simulink model "Simple"  (Simulink 7.4)
settings: Solver=ode45  StartTime=0.0  StopTime=80  RelTol=1e-3
settings Model: Creator=Lluís  LastModifiedBy=Lluís

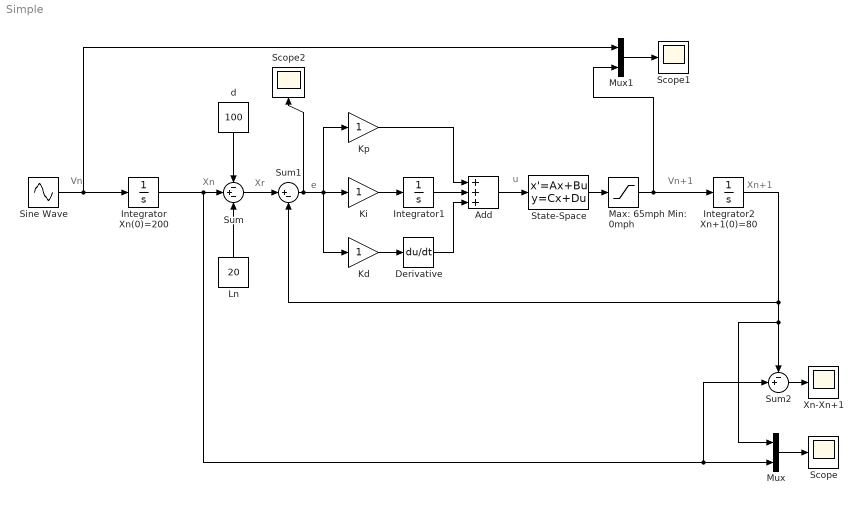
== system Simple ==
  note: Vn
  note: Xn
  note: Xr
  note: e
  note: u
  note: Vn+1
  note: Xn+1
  Add : Sum  Inputs=+++  OutDataType=fixdt(1, 16)  OutScaling=2^-10
  Derivative : Derivative
  Integrator Xn(0)=200 : Integrator  InitialCondition=200
  Integrator1 : Integrator
  Integrator2 Xn+1(0)=80 : Integrator  InitialCondition=80
  Kd : Gain  ParameterDataType=fixdt(1, 16)  ParameterScaling=2^0  OutDataType=fixdt(1, 16)  OutScaling=2^0
  Ki : Gain  ParameterDataType=fixdt(1, 16)  ParameterScaling=2^0  OutDataType=fixdt(1, 16)  OutScaling=2^0
  Kp : Gain  ParameterDataType=fixdt(1, 16)  ParameterScaling=2^0  OutDataType=fixdt(1, 16)  OutScaling=2^0
  Ln : Constant  Value=20  OutDataType=fixdt(1, 16)  OutScaling=2^0
  Max: 65mph Min: 0mph : Saturate  UpperLimit=95.33  LowerLimit=0  OutDataType=fixdt(1, 16)  OutScaling=2^0
  Mux : Mux  Inputs=2
  Mux1 : Mux  Inputs=2
  Scope : Scope
  Scope1 : Scope
      settings: SaveName=data2  DataFormat=Array
  Scope2 : Scope
      settings: SaveName=ScopeData3
  Sine Wave : Sin  Amplitude=22  Bias=22  Frequency=pi()/5  Phase=pi()/2  Samples=10  SampleTime=0  Offset=0
  State-Space : StateSpace  A=0  D=0  X0=44
  Sum : Sum  Inputs=-+-  OutDataType=fixdt(1, 16)  OutScaling=2^0
  Sum1 : Sum  Inputs=|+-  OutDataType=fixdt(1, 16)  OutScaling=2^0
  Sum2 : Sum  Inputs=-+|  OutDataType=fixdt(1, 16)  OutScaling=2^0
  Xn-Xn+1 : Scope
      settings: SaveName=data  DataFormat=Array
  d : Constant  Value=100  OutDataType=fixdt(1, 16)  OutScaling=2^0
  wires:
  Sine Wave/1 -> Integrator Xn(0)=200/1, Mux1/1
  d/1 -> Sum/1
  Ln/1 -> Sum/3
  Sum/1 -> Sum1/1
  Sum1/1 -> Kp/1, Kd/1, Ki/1, Scope2/1
  Ki/1 -> Integrator1/1
  Kd/1 -> Derivative/1
  State-Space/1 -> Max: 65mph Min: 0mph/1
  Integrator2 Xn+1(0)=80/1 -> Sum2/1, Mux/1, Sum1/2
  Integrator1/1 -> Add/2
  Add/1 -> State-Space/1
  Kp/1 -> Add/1
  Derivative/1 -> Add/3
  Max: 65mph Min: 0mph/1 -> Mux1/2, Integrator2 Xn+1(0)=80/1
  Integrator Xn(0)=200/1 -> Sum/2, Mux/2, Sum2/2
  Sum2/1 -> Xn-Xn+1/1
  Mux/1 -> Scope/1
  Mux1/1 -> Scope1/1
